simulink model "iot_ann"  (R2024b)
settings: Solver=VariableStepAuto  StartTime=0.0  StopTime=20  RelTol=1e-3
libraries: sldrtlib x4
settings Model: Creator=KIIT  LastModifiedBy=KIIT

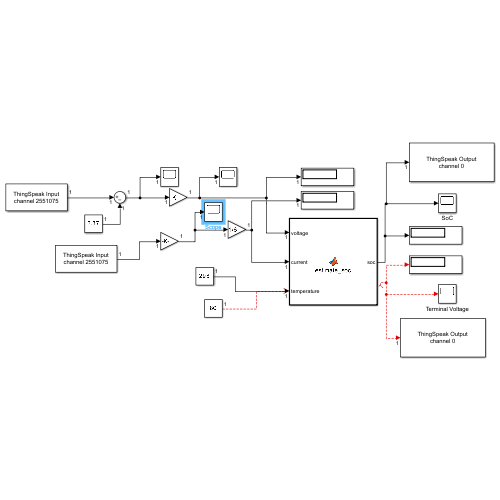
[thumbnail: Simulink's stored preview of the top-level diagram]
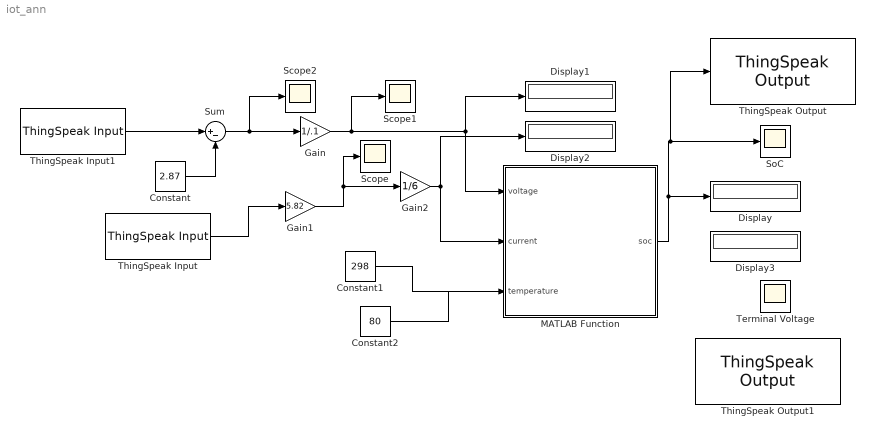
== system iot_ann ==
  Constant : Constant  Value=2.87
  Constant1 : Constant  Value=298
  Constant2 : Constant  Value=80
  Display{,1..3} (4 alike) : Display
  Gain : Gain  Gain=1/.1
  Gain1 : Gain  Gain=5.82
  Gain2 : Gain  Gain=1/6
  MATLAB Function : MATLAB Function  TreatAsAtomicUnit=on
  Scope : Scope
  Scope1 : Scope
  Scope2 : Scope
  SoC : Scope
  Sum : Sum  Inputs=|+-
  Terminal Voltage : Scope
  ThingSpeak Input : sldrtlib/Internet of Things/ThingSpeak Input  DrvAddress=2551075  DrvOptions=[0 20 32 52 66 68 87 86 86 85 65 83 66 79 77 78 90 90 97 112 105 46 116 104 105 110 103 115 112 101 97 107 46 99 111 109 0 0 0 0 0 0 0 0 0 0 0 0 0 0 0 0 0 0 0 0 0 0 0 0 0 0 0 0 0 0 0 0 0 0 0 0 0 0 0 0 0 0 0 0 0 0 0 0 0 0 0 0 0 0 0 0 0 0 0 0 0 0 0 0 0 0 0 0 0 0 0 0 0 0 0 0 0 0 0 0 0 0 0 0 0 0 0 0 0 0 0 0 0 0 0 0 0 0 0 0 0 0 0 0 0 0 0 0 0 0 0 0 0 0 0 0 0 0 0 0 0 0 0 0 0 0 0 0 0 0 0 0 0 0 0 0 0 0 0 0 0 0 0 0 0 0 0 0 0 0 0 0 0 0 0 0 0 0 0 0 0 0 0 0 0 0 0 0 0 0 0 0 0 0 0 0 0 0 0 0 0 0 0 0 0 0 0 0 0 0 0 0 0 0 0 0 0 0 0 0 0 0 0 0 0 0 0 0 0 0 0 0 0 0 0 0 0 0 0 0]  SampleTime=2  MaxMissedTicks=10000  ShowMissedTicks=off  YieldWhenWaiting=off  ChannelFields=2  OptParam=0  DataTypeStr=double
  ThingSpeak Input1 : sldrtlib/Internet of Things/ThingSpeak Input  DrvAddress=2551075  DrvOptions=[0 20 52 66 68 87 86 86 85 65 83 66 79 77 78 90 90 87 97 112 105 46 116 104 105 110 103 115 112 101 97 107 46 99 111 109 0 0 0 0 0 0 0 0 0 0 0 0 0 0 0 0 0 0 0 0 0 0 0 0 0 0 0 0 0 0 0 0 0 0 0 0 0 0 0 0 0 0 0 0 0 0 0 0 0 0 0 0 0 0 0 0 0 0 0 0 0 0 0 0 0 0 0 0 0 0 0 0 0 0 0 0 0 0 0 0 0 0 0 0 0 0 0 0 0 0 0 0 0 0 0 0 0 0 0 0 0 0 0 0 0 0 0 0 0 0 0 0 0 0 0 0 0 0 0 0 0 0 0 0 0 0 0 0 0 0 0 0 0 0 0 0 0 0 0 0 0 0 0 0 0 0 0 0 0 0 0 0 0 0 0 0 0 0 0 0 0 0 0 0 0 0 0 0 0 0 0 0 0 0 0 0 0 0 0 0 0 0 0 0 0 0 0 0 0 0 0 0 0 0 0 0 0 0 0 0 0 0 0 0 0 0 0 0 0 0 0 0 0 0 0 0 0 0 0 0]  SampleTime=2  MaxMissedTicks=10000  ShowMissedTicks=off  YieldWhenWaiting=off  ChannelFields=1  OptParam=0  DataTypeStr=double
  ThingSpeak Output : sldrtlib/Internet of Things/ThingSpeak Output  DrvAddress=0  DrvOptions=[1 20 0 0 0 0 0 0 0 0 0 0 0 0 0 0 0 0 97 112 105 46 116 104 105 110 103 115 112 101 97 107 46 99 111 109 0 0 0 0 0 0 0 0 0 0 0 0 0 0 0 0 0 0 0 0 0 0 0 0 0 0 0 0 0 0 0 0 0 0 0 0 0 0 0 0 0 0 0 0 0 0 0 0 0 0 0 0 0 0 0 0 0 0 0 0 0 0 0 0 0 0 0 0 0 0 0 0 0 0 0 0 0 0 0 0 0 0 0 0 0 0 0 0 0 0 0 0 0 0 0 0 0 0 0 0 0 0 0 0 0 0 0 0 0 0 0 0 0 0 0 0 0 0 0 0 0 0 0 0 0 0 0 0 0 0 0 0 0 0 0 0 0 0 0 0 0 0 0 0 0 0 0 0 0 0 0 0 0 0 0 0 0 0 0 0 0 0 0 0 0 0 0 0 0 0 0 0 0 0 0 0 0 0 0 0 0 0 0 0 0 0 0 0 0 0 0 0 0 0 0 0 0 0 0 0 0 0 0 0 0 0 0 0 0 0 0 0 0 0 0 0 0 0 0 0]  SampleTime=0.1  MaxMissedTicks=10  ShowMissedTicks=off  YieldWhenWaiting=off  ChannelFields=1  OptParam=0  InitialValue=[]  FinalValue=[]
  ThingSpeak Output1 : sldrtlib/Internet of Things/ThingSpeak Output  DrvAddress=0  DrvOptions=[1 20 0 0 0 0 0 0 0 0 0 0 0 0 0 0 0 0 97 112 105 46 116 104 105 110 103 115 112 101 97 107 46 99 111 109 0 0 0 0 0 0 0 0 0 0 0 0 0 0 0 0 0 0 0 0 0 0 0 0 0 0 0 0 0 0 0 0 0 0 0 0 0 0 0 0 0 0 0 0 0 0 0 0 0 0 0 0 0 0 0 0 0 0 0 0 0 0 0 0 0 0 0 0 0 0 0 0 0 0 0 0 0 0 0 0 0 0 0 0 0 0 0 0 0 0 0 0 0 0 0 0 0 0 0 0 0 0 0 0 0 0 0 0 0 0 0 0 0 0 0 0 0 0 0 0 0 0 0 0 0 0 0 0 0 0 0 0 0 0 0 0 0 0 0 0 0 0 0 0 0 0 0 0 0 0 0 0 0 0 0 0 0 0 0 0 0 0 0 0 0 0 0 0 0 0 0 0 0 0 0 0 0 0 0 0 0 0 0 0 0 0 0 0 0 0 0 0 0 0 0 0 0 0 0 0 0 0 0 0 0 0 0 0 0 0 0 0 0 0 0 0 0 0 0 0]  SampleTime=0.1  MaxMissedTicks=10  ShowMissedTicks=off  YieldWhenWaiting=off  ChannelFields=1  OptParam=0  InitialValue=[]  FinalValue=[]
  wires:
  ThingSpeak Input/1 -> Gain1/1
  Gain/1 -> Scope1/1, MATLAB Function/1(voltage), Display1/1
  Gain1/1 -> Scope/1, Gain2/1
  ThingSpeak Input1/1 -> Sum/1
  Constant/1 -> Sum/2
  Sum/1 -> Scope2/1, Gain/1
  Constant1/1 -> MATLAB Function/3(temperature)
  Constant2/1 -> ?
  Gain2/1 -> MATLAB Function/2(current), Display2/1
  MATLAB Function/1(soc) -> ThingSpeak Output/1, SoC/1, Display/1
  ? -> Display3/1, ThingSpeak Output1/1, Terminal Voltage/1

== matlab function iot_ann/MATLAB Function ==
  data: voltage input; soc output; current input; temperature input
function soc = estimate_soc(voltage, current, temperature)
%#codegen

    persistent W1 b1 W2 b2;

    % Load ANN Parameters only once
    if isempty(W1)
        coder.load('ann_parameters.mat', 'W1', 'b1', 'W2', 'b2');
    end

    % === Normalize Inputs (Ensure Consistency with Training) ===
    voltage_min = 3.0; voltage_max = 4.2; 
    current_min = 0.1; current_max = 5.0;
    temp_min = 20; temp_max = 50;

    v_norm = (voltage - voltage_min) / (voltage_max - voltage_min);
    i_norm = (current - current_min) / (current_max - current_min);
    t_norm = (temperature - temp_min) / (temp_max - temp_min);

    % === Forward Propagation (ANN Calculation) ===
    x = [v_norm; i_norm; t_norm];  % Input vector
    
    % Hidden layer computation (ReLU activation)
    hidden_layer = max(0, W1 * x + b1);

    % Output layer computation (Linear activation)
    soc = W2 * hidden_layer + b2;

    % Ensure SoC is within valid range [0,1]
    soc = min(max(soc, 0), 1);
end
